simulink model "Eric_Malmquist_Sim1"  (R2020b)
settings: Solver=FixedStepAuto  StartTime=0.0  StopTime=10.0  RelTol=1e-3
settings Model: Creator=malmquie  LastModifiedBy=Eric Malmquist
settings OptimizationCC: OptimizeBlockIOStorage=off  ZeroExternalMemoryAtStartup=off  ZeroInternalMemoryAtStartup=off  OptimizeDataStoreBuffers=off  BusAssignmentInplaceUpdate=off
settings DebuggingCC: SFUnexpectedBacktrackingDiag=warning  SFNoUnconditionalDefaultTransitionDiag=warning
settings SFSimCC: CustomCodeUndefinedFunction=UseInterfaceOnly
settings RTWCC: GenerateReport=on  BuildConfiguration=Debug  LaunchReport=on  TargetLang=C++
settings CodeAppCC: ForceParamTrailComments=on  MATLABSourceComments=on  EnableCustomComments=on
settings GRTTargetCC: TargetLangStandard=C++03 (ISO)  CombineSignalStateStructs=on  CodeInterfacePackaging=C++ class  SupportVariableSizeSignals=on  MultiInstanceErrorCode=Warning

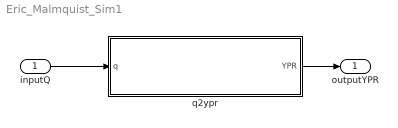
== system Eric_Malmquist_Sim1 ==
  inputQ : Inport  PortDimensions=4
  q2ypr : Subsystem
  outputYPR : Outport  PortDimensions=3
  wires:
  inputQ/1 -> q2ypr/1(q)
  q2ypr/1(YPR) -> outputYPR/1

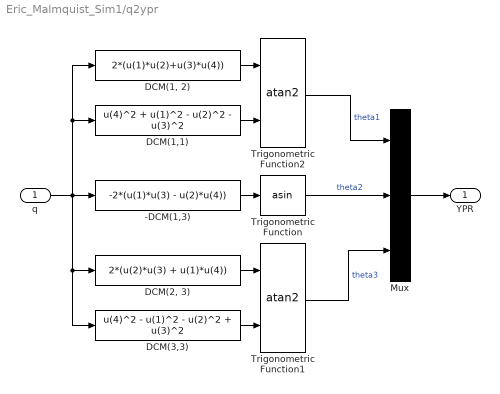
== system Eric_Malmquist_Sim1/q2ypr ==
  q : Inport
  -DCM(1,3) : Fcn  Expr=-2*(u(1)*u(3) - u(2)*u(4))
  "DCM(1, 2)" : Fcn  Expr=2*(u(1)*u(2)+u(3)*u(4))
  DCM(1,1) : Fcn  Expr=u(4)^2 + u(1)^2 - u(2)^2 - u(3)^2
  "DCM(2, 3)" : Fcn  Expr=2*(u(2)*u(3) + u(1)*u(4))
  DCM(3,3) : Fcn  Expr=u(4)^2 - u(1)^2 - u(2)^2 + u(3)^2
  Mux : Mux  Inputs=3
  Trigonometric Function : Trigonometry  Operator=asin
  Trigonometric Function1 : Trigonometry  Operator=atan2
  Trigonometric Function2 : Trigonometry  Operator=atan2
  YPR : Outport  VectorParamsAs1DForOutWhenUnconnected=off
  wires:
  Mux/1 -> YPR/1
  -DCM(1,3)/1 -> Trigonometric Function/1
  Trigonometric Function/1 -> Mux/2  "theta2"
  Trigonometric Function1/1 -> Mux/3  "theta3"
  "DCM(2, 3)"/1 -> Trigonometric Function1/1
  DCM(3,3)/1 -> Trigonometric Function1/2
  q/1 -> DCM(3,3)/1, "DCM(2, 3)"/1, "DCM(1, 2)"/1, DCM(1,1)/1, -DCM(1,3)/1
  Trigonometric Function2/1 -> Mux/1  "theta1"
  DCM(1,1)/1 -> Trigonometric Function2/2
  "DCM(1, 2)"/1 -> Trigonometric Function2/1
